simulink model "send_nad"  (R2019b)
settings: Solver=FixedStepAuto  StartTime=0.0  StopTime=10.0  RelTol=1e-3
PreLoadFcn:
  | fprintf(1, '[PreLoadFcn] Load send_nad_sample_inputs.mat\n');
  | load('send_nad_sample_inputs')
model workspace (MAT data in the model file):
  ED247Configuration(1).name = 'Signal00'
  ED247Configuration(1).direction = 'OUT'
  ED247Configuration(1).type = 'uint8'
  ED247Configuration(1).dimensions = 1
  ED247Configuration(1).width = 1
  ED247Configuration(1).size = 1
  ED247Configuration(1).sample_time = 0.00999999977648
  ED247Configuration(1).validity_duration = 0
  ED247Configuration(1).signal_type = 'NAD'
  ED247Configuration(1).sample_size = 1
  ED247Configuration(2).name = 'Signal01'
  ED247Configuration(2).direction = 'OUT'
  ED247Configuration(2).type = 'uint8'
  ED247Configuration(2).dimensions = 1
  ED247Configuration(2).width = 1
  ED247Configuration(2).size = 1
  ED247Configuration(2).sample_time = 0.00999999977648
  ED247Configuration(2).validity_duration = 0
  ED247Configuration(2).signal_type = 'NAD'
  ED247Configuration(2).sample_size = 1
  ED247Configuration(3).name = 'Signal10'
  ED247Configuration(3).direction = 'OUT'
  ED247Configuration(3).type = 'uint8'
  ED247Configuration(3).dimensions = 1
  ED247Configuration(3).width = 1
  ED247Configuration(3).size = 1
  ED247Configuration(3).sample_time = 0.00999999977648
  ED247Configuration(3).validity_duration = 0
  ED247Configuration(3).signal_type = 'NAD'
  ED247Configuration(3).sample_size = 1
  ED247Configuration(4).name = 'Signal11'
  ED247Configuration(4).direction = 'OUT'
  ED247Configuration(4).type = 'single'
  ED247Configuration(4).dimensions = 2
  ED247Configuration(4).width = 4
  ED247Configuration(4).size = [2 2]
  ED247Configuration(4).sample_time = 0.00999999977648
  ED247Configuration(4).validity_duration = 0
  ED247Configuration(4).signal_type = 'NAD'
  ED247Configuration(4).sample_size = 16
libraries: lib_ed247 x2
settings Model: EnablePacing=on  Creator=odufour  LastModifiedBy=odufour
settings DataIOCC: ExternalInput=ds  LoadExternalInput=on
settings OptimizationCC: DefaultParameterBehavior=Inlined  EnhancedBackFolding=on  PassReuseOutputArgsAs=Individual arguments  ZeroExternalMemoryAtStartup=off  ZeroInternalMemoryAtStartup=off  OptimizeBlockOrder=speed  DifferentSizesBufferReuse=on  OptimizationCustomize=off  EfficientTunableParamExpr=on
settings DebuggingCC: ParameterTunabilityLossMsg=error
settings SFSimCC: MATLABDynamicMemAlloc=off
settings RTWCC: SystemTargetFile=ert.tlc  GenCodeOnly=on  TemplateMakefile=ert_default_tmf  GenerateReport=on  IncludeHyperlinkInReport=on  GenerateTraceInfo=on  GenerateTraceReport=on  GenerateTraceReportSl=on  GenerateTraceReportSf=on  GenerateTraceReportEml=on
settings CodeAppCC: ForceParamTrailComments=on  IgnoreCustomStorageClasses=off  OperatorAnnotations=on  SimulinkDataObjDesc=on  SFDataObjDesc=on  InsertBlockDesc=on
settings ERTTargetCC: TargetLangStandard=C99 (ISO)  GenerateSampleERTMain=on  InlinedParameterPlacement=NonHierarchical  ERTCustomFileTemplate=example_file_process.tlc

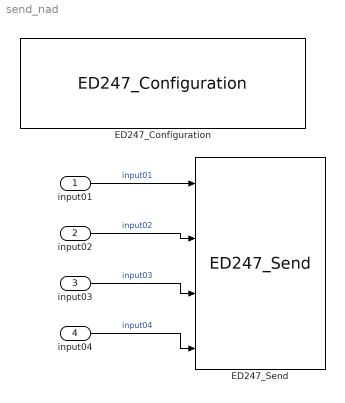
== system send_nad ==
  input01 : Inport  OutDataTypeStr=uint8  SampleTime=0.5
  input02 : Inport  Port=2  OutDataTypeStr=uint8  SampleTime=0.5
  input03 : Inport  Port=3  OutDataTypeStr=uint8  SampleTime=0.5
  input04 : Inport  Port=4  OutDataTypeStr=single  PortDimensions=[2,2]  SampleTime=0.5
  ED247_Configuration : lib_ed247/ED247_Configuration  configurationFilename='ecic_func_exchange_nad_uc_main.xml'  enableLog=off  logFilename=''
      settings: SourceProductName=Airbus ED247
  ED247_Send : lib_ed247/ED247_Send  enable_refresh=off  show_port_labels=on
      settings: SourceProductName=Airbus ED247
  wires:
  input01/1 -> ED247_Send/1  "input01"
  input02/1 -> ED247_Send/2  "input02"
  input03/1 -> ED247_Send/3  "input03"
  input04/1 -> ED247_Send/4  "input04"
